simulink model "Task2"  (R2019a)
settings: Solver=VariableStepAuto  StartTime=0.0  StopTime=10.0  RelTol=1e-3
settings Model: Creator=Acer  LastModifiedBy=Acer

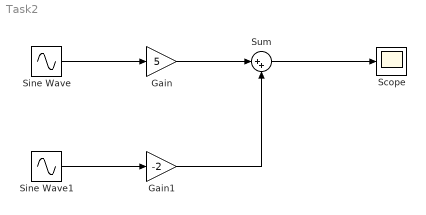
== system Task2 ==
  Gain : Gain  Gain=5
  Gain1 : Gain  Gain=-2
  Scope : Scope
  Sine Wave : Sin  Phase=pi/2  SampleTime=0
  Sine Wave1 : Sin  SampleTime=0
  Sum : Sum  Inputs=|++
  wires:
  Sine Wave/1 -> Gain/1
  Sine Wave1/1 -> Gain1/1
  Gain/1 -> Sum/1
  Gain1/1 -> Sum/2
  Sum/1 -> Scope/1
